simulink model "lab_final_1"  (R2024b)
settings: Solver=VariableStepAuto  StartTime=0.0  StopTime=10  RelTol=1e-3
values from neighbouring files (symbols this model uses):
  A = [0 1 0 0 ... (first row only)    [code_cte_small.m]    (also in lab1.m)
  Afcc = inv(T) * A * T    [code_cte_small.m]    (also in lab1.m)
  Afco = inv(Q)*A*Q    [code_cte_small.m]    (also in lab1.m)
  B = [0 ... (first row only)    [code_cte_small.m]    (also in lab1.m)
  Bfcc = inv(T) * B    [code_cte_small.m]    (also in lab1.m)
  Bfco = inv(Q) * B    [code_cte_small.m]    (also in lab1.m)
  C = [1 0 0 0]    [code_cte_small.m]    (also in lab1.m)
  Cfcc = C * T    [code_cte_small.m]    (also in lab1.m)
  Cfco = C * Q    [code_cte_small.m]    (also in lab1.m)
  E = [0 ... (first row only)    [code_cte_small.m]    (also in lab1.m)
  Efcc = inv(T)*E    [code_cte_small.m]    (also in lab1.m)
  Efco = inv(Q) * E    [code_cte_small.m]    (also in lab1.m)
  F1 = ((k2 + k1)/m)*xb + ((M/m) - 1)*g*sin(thetaop)    [code_cte_small.m]    (also in lab1.m)
  k_obs_F_matriz = inv(matriz_P_f)*k_cachuchita_f'    [code_cte_small.m]    (also in lab1.m)
  KA = [-19.21, 9.68, 4.10, -15.739]    [code_cte_small.m]    (also in lab1.m = [-15.3759, -7.2896182, -45.976447, -15.168131])
  KAfcc = [-29798.327,25528.529, 7395.9961,14.998605]    [code_cte_small.m]    (also in lab1.m)
  KAfco = [-3.2913256, 1568.6046, -768661.08, 376589940.0 ]    [code_cte_small.m]    (also in lab1.m)
  kiA = -24.76    [code_cte_small.m]    (also in lab1.m = -151.09413)
  kiAfcc = [-151.09413]    [code_cte_small.m]    (also in lab1.m)
  kiAfco = [-151.09413]    [code_cte_small.m]    (also in lab1.m)
  xb = 0.5    [code_cte_small.m]    (also in lab1.m)
settings Model: Creator=Acer  LastModifiedBy=Acer

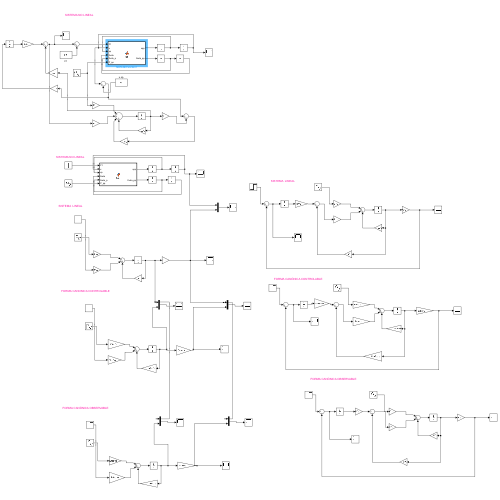
[thumbnail: Simulink's stored preview of the top-level diagram]
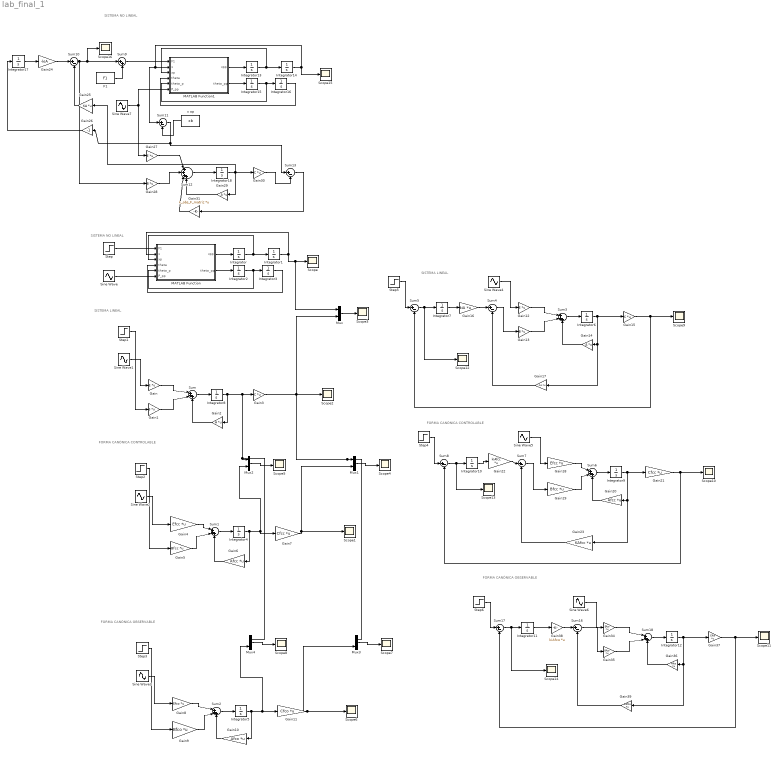
== system lab_final_1 ==
  note: SISTEMA LINEAL
  note: SISTEMA NO LINEAL
  note: FORMA CANÓNICA CONTROLABLE
  note: FORMA CANÓNICA OBSERVABLE
  note: SISTEMA LINEAL
  note: FORMA CANÓNICA CONTROLABLE
  note: FORMA CANÓNICA OBSERVABLE
  note: SISTEMA NO LINEAL
  F1 : Constant  Value=F1
  Gain : Gain  Gain=E  Multiplication=Matrix(K*u)
  Gain1 : Gain  Gain=B  Multiplication=Matrix(K*u)
  Gain10 : Gain  Gain=Afco  Multiplication=Matrix(K*u)
  Gain11 : Gain  Gain=Cfco  Multiplication=Matrix(K*u)
  Gain12 : Gain  Gain=E  Multiplication=Matrix(K*u)
  Gain13 : Gain  Gain=B  Multiplication=Matrix(K*u)
  Gain14 : Gain  Gain=A  Multiplication=Matrix(K*u)
  Gain15 : Gain  Gain=C  Multiplication=Matrix(K*u)
  Gain16 : Gain  Gain=kiA  Multiplication=Matrix(K*u)
  Gain17 : Gain  Gain=KA  Multiplication=Matrix(K*u)
  Gain18 : Gain  Gain=Efcc  Multiplication=Matrix(K*u)
  Gain19 : Gain  Gain=Bfcc  Multiplication=Matrix(K*u)
  Gain2 : Gain  Gain=A  Multiplication=Matrix(K*u)
  Gain20 : Gain  Gain=Afcc  Multiplication=Matrix(K*u)
  Gain21 : Gain  Gain=Cfcc  Multiplication=Matrix(K*u)
  Gain22 : Gain  Gain=kiAfcc  Multiplication=Matrix(K*u)
  Gain23 : Gain  Gain=KAfcc  Multiplication=Matrix(K*u)
  Gain24 : Gain  Gain=-kiA
  Gain25 : Gain  Gain=KA  Multiplication=Matrix(K*u)
  Gain26 : Gain  Gain=-1
  Gain27 : Gain  Gain=E  Multiplication=Matrix(K*u)
  Gain28 : Gain  Gain=B  Multiplication=Matrix(K*u)
  Gain29 : Gain  Gain=A  Multiplication=Matrix(K*u)
  Gain3 : Gain  Gain=C  Multiplication=Matrix(K*u)
  Gain30 : Gain  Gain=C  Multiplication=Matrix(K*u)
  Gain31 : Gain  Gain=k_obs_F_matriz  Multiplication=Matrix(K*u)
  Gain34 : Gain  Gain=Efco  Multiplication=Matrix(K*u)
  Gain35 : Gain  Gain=Bfco  Multiplication=Matrix(K*u)
  Gain36 : Gain  Gain=Afco  Multiplication=Matrix(K*u)
  Gain37 : Gain  Gain=Cfco  Multiplication=Matrix(K*u)
  Gain38 : Gain  Gain=kiAfco  Multiplication=Matrix(K*u)
  Gain39 : Gain  Gain=KAfco  Multiplication=Matrix(K*u)
  Gain4 : Gain  Gain=Efcc  Multiplication=Matrix(K*u)
  Gain5 : Gain  Gain=Bfcc  Multiplication=Matrix(K*u)
  Gain6 : Gain  Gain=Afcc  Multiplication=Matrix(K*u)
  Gain7 : Gain  Gain=Cfcc  Multiplication=Matrix(K*u)
  Gain8 : Gain  Gain=Efco  Multiplication=Matrix(K*u)
  Gain9 : Gain  Gain=Bfco  Multiplication=Matrix(K*u)
  Integrator{,1..18} (19 alike) : Integrator
  MATLAB Function : MATLAB Function  TreatAsAtomicUnit=on
  MATLAB Function1 : MATLAB Function  TreatAsAtomicUnit=on
  Mux{,1..4} (5 alike) : Mux  Inputs=2
  Scope{,1..16} (17 alike) : Scope
  Sine Wave{,1..6} (7 alike) : Sin  Frequency=5  SampleTime=0
  Sine Wave7 : Sin  Amplitude=0  Frequency=0  SampleTime=0
  Step{,1..6} (7 alike) : Step  Time=0  SampleTime=0
  Sum{,1..3,6,18} (6 alike) : Sum  Inputs=|+++
  Sum{4..5,7..8,10..11,13,16..17} (9 alike) : Sum  Inputs=|+-
  Sum12 : Sum  Inputs=|++++
  Sum9 : Sum  Inputs=|++
  x op : Constant  Value=xb
  wires:
  MATLAB Function/1(xpp) -> Integrator/1
  Integrator/1 -> Integrator1/1, MATLAB Function/3(xp)
  Integrator1/1 -> MATLAB Function/2(x), Mux/1, Scope/1
  MATLAB Function/2(theta_pp) -> Integrator2/1
  Integrator2/1 -> Integrator3/1, MATLAB Function/5(theta_p)
  Integrator3/1 -> MATLAB Function/4(theta)
  Sine Wave/1 -> MATLAB Function/6(P_pp)
  Step/1 -> MATLAB Function/1(F1)
  Step1/1 -> Gain1/1
  Sine Wave1/1 -> Gain/1
  Gain/1 -> Sum/1
  Gain1/1 -> Sum/2
  Sum/1 -> Integrator8/1
  Gain2/1 -> Sum/3
  Integrator8/1 -> Gain2/1, Mux4/1, Mux2/1, Gain3/1
  Gain3/1 -> Mux3/1, Mux1/1, Scope2/1, Mux/2
  Mux/1 -> Scope3/1
  Gain7/1 -> Mux1/2, Scope1/1
  Integrator4/1 -> Mux2/2, Gain7/1, Gain6/1
  Gain6/1 -> Sum1/3
  Sum1/1 -> Integrator4/1
  Gain5/1 -> Sum1/2
  Gain4/1 -> Sum1/1
  Step2/1 -> Gain5/1
  Sine Wave2/1 -> Gain4/1
  Mux1/1 -> Scope4/1
  Mux2/1 -> Scope5/1
  Mux4/1 -> Scope8/1
  Mux3/1 -> Scope7/1
  Sine Wave3/1 -> Gain8/1
  Step3/1 -> Gain9/1
  Gain8/1 -> Sum2/1
  Gain9/1 -> Sum2/2
  Sum2/1 -> Integrator5/1
  Gain10/1 -> Sum2/3
  Integrator5/1 -> Gain10/1, Gain11/1, Mux4/2
  Gain11/1 -> Mux3/2, Scope6/1
  Integrator6/1 -> Gain15/1, Gain17/1, Gain14/1
  Gain14/1 -> Sum3/3
  Sum3/1 -> Integrator6/1
  Gain13/1 -> Sum3/2
  Gain12/1 -> Sum3/1
  Sine Wave4/1 -> Gain12/1
  Step5/1 -> Sum5/1
  Sum5/1 -> Scope12/1, Integrator7/1
  Integrator7/1 -> Gain16/1
  Gain16/1 -> Sum4/1
  Gain17/1 -> Sum4/2
  Gain15/1 -> Sum5/2, Scope9/1
  Sum4/1 -> Gain13/1
  Sum7/1 -> Gain19/1
  Gain21/1 -> Scope10/1, Sum8/2
  Gain23/1 -> Sum7/2
  Gain22/1 -> Sum7/1
  Integrator10/1 -> Gain22/1
  Sum8/1 -> Scope13/1, Integrator10/1
  Step4/1 -> Sum8/1
  Sine Wave5/1 -> Gain18/1
  Gain18/1 -> Sum6/1
  Gain19/1 -> Sum6/2
  Sum6/1 -> Integrator9/1
  Gain20/1 -> Sum6/3
  Integrator9/1 -> Gain20/1, Gain23/1, Gain21/1
  Gain34/1 -> Sum18/1
  Sum16/1 -> Gain35/1
  Sum18/1 -> Integrator12/1
  Gain38/1 -> Sum16/1
  Sum17/1 -> Scope14/1, Integrator11/1
  Step6/1 -> Sum17/1
  Gain35/1 -> Sum18/2
  Integrator12/1 -> Gain37/1, Gain39/1, Gain36/1
  Gain37/1 -> Sum17/2, Scope11/1
  Gain39/1 -> Sum16/2
  Sine Wave6/1 -> Gain34/1
  Integrator11/1 -> Gain38/1
  Gain36/1 -> Sum18/3
  Sine Wave7/1 -> Gain27/1, MATLAB Function1/6(P_pp)
  Integrator16/1 -> MATLAB Function1/4(theta)
  Integrator15/1 -> MATLAB Function1/5(theta_p), Integrator16/1
  MATLAB Function1/2(theta_pp) -> Integrator15/1
  Integrator14/1 -> Scope15/1, MATLAB Function1/2(x), Sum11/1
  Integrator13/1 -> MATLAB Function1/3(xp), Integrator14/1
  MATLAB Function1/1(xpp) -> Integrator13/1
  Sum9/1 -> MATLAB Function1/1(F1)
  F1/1 -> Sum9/2
  Sum10/1 -> Scope16/1, Sum9/1, Gain28/1
  Gain24/1 -> Sum10/1
  Integrator17/1 -> Gain24/1
  Gain25/1 -> Sum10/2
  Gain26/1 -> Integrator17/1
  x op/1 -> Sum11/2
  Gain27/1 -> Sum12/1
  Gain28/1 -> Sum12/2
  Gain29/1 -> Sum12/4
  Sum12/1 -> Integrator18/1
  Integrator18/1 -> Gain25/1, Gain29/1, Gain30/1
  Gain30/1 -> Sum13/2
  Sum11/1 -> Sum13/1, Gain26/1
  Gain31/1 -> Sum12/3
  Sum13/1 -> Gain31/1

== matlab function lab_final_1/MATLAB Function1 ==
  data: F1 input; xpp output; x input; xp input; theta input; theta_p input; P_pp input; theta_pp output
function [xpp,theta_pp] = fcn(F1,x,xp, theta,theta_p, P_pp)
k1 = 323;     % N/m
k2 = 556;     % N/m
b1 = 432;   % Ns/m
b2 = 23;   % Ns/m
M  = 50;   % kg
m  = 43;   % kg
g  = 9.81;  % m/s^2
L  = 1;   % m
xpp= (F1-xp*(b1+b2)-x*(k1+k2)+M*g*sin(theta))/m
theta_pp= (-P_pp+((b2+b1)/m)*xp+((k2+k1)/m)*x+((-M/m)-1)*g*sin(theta)-F1)/L;

== matlab function lab_final_1/MATLAB Function ==
  data: F1 input; xpp output; x input; xp input; theta input; theta_p input; P_pp input; theta_pp output
function [xpp,theta_pp] = fcn(F1,x,xp, theta,theta_p, P_pp)
k1 = 323;     % N/m
k2 = 556;     % N/m
b1 = 432;   % Ns/m
b2 = 23;   % Ns/m
M  = 50;   % kg
m  = 43;   % kg
g  = 9.81;  % m/s^2
L  = 1;   % m
xpp= (F1-xp*(b1+b2)-x*(k1+k2)+M*g*sin(theta))/m
theta_pp= (-P_pp+((b2+b1)/m)*xp+((k2+k1)/m)*x+((-M/m)-1)*g*sin(theta)-F1)/L;
